simulink library "powerEstimate"  (R2018a)
settings: Solver=VariableStepAuto  StartTime=0.0  StopTime=10.0  RelTol=1e-3
settings Model: Creator=mitch  LastModifiedBy=mitch

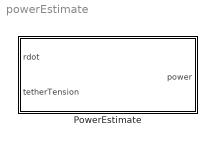
== system powerEstimate ==
  PowerEstimate : Subsystem

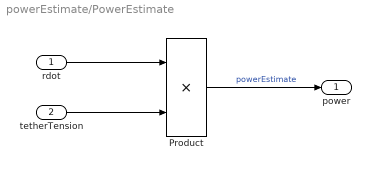
== system powerEstimate/PowerEstimate ==
  rdot : Inport
  tetherTension : Inport  Port=2
  Product : Product
  power : Outport
  wires:
  Product/1 -> power/1  "powerEstimate"
  rdot/1 -> Product/1
  tetherTension/1 -> Product/2
